simulink model "randomVelToLeader"  (R2018b)
settings: Solver=VariableStepAuto  StartTime=0.0  StopTime=inf  RelTol=1e-3
undefined symbols (not defined in the file or in its folder): Angular, Linear
libraries: robotlib x2
settings Model: Creator=ckreienk  LastModifiedBy=ckreienk

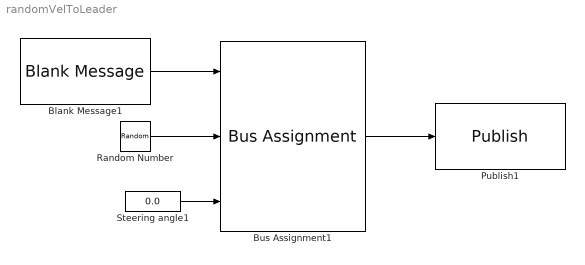
== system randomVelToLeader ==
  Blank Message1 : robotlib/Blank Message  messageClass=Message  entityType=geometry_msgs/Twist  messageType=geometry_msgs/Twist  SampleTime=inf
      settings: SourceProductBaseCode=RO
  Bus Assignment1 : BusAssignment  AssignedSignals=Linear.X,Angular.Z
  Publish1 : robotlib/Publish  topicSource=Select from ROS network  topic=/leadVehicle/cmd_vel  messageType=geometry_msgs/Twist  messageQueueLength=1
      settings: SourceProductBaseCode=RO
  Random Number : RandomNumber  Mean=4  Variance=5  SampleTime=1
  Steering angle1 : Constant  Value=0.0
  wires:
  Steering angle1/1 -> Bus Assignment1/3
  Random Number/1 -> Bus Assignment1/2
  Blank Message1/1 -> Bus Assignment1/1
  Bus Assignment1/1 -> Publish1/1
